simulink model "simulink_ascent_model_variable_mass_displayorganization"  (R2020a)
settings: Solver=FixedStepAuto  StartTime=0.0  StopTime=36000  FixedStep=dt  RelTol=1e-5
values from neighbouring files (symbols this model uses):
  altimeter_noise_gain = 0    [ascent_model_variable_mass.m]
  arm_tolerance = 1000    [ascent_model_variable_mass.m]
  atmo_density_noise_gain = 0    [ascent_model_variable_mass.m]
  atmo_pres_noise_gain = 0    [ascent_model_variable_mass.m]
  atmo_temp_noise_gain = 0    [ascent_model_variable_mass.m]
  burst_volume = balloon_parameters.spec.volume_burst.value    [ascent_model_variable_mass.m]
  Cd = balloon_parameters.spec.drag_coefficient    [ascent_model_variable_mass.m]
  continuous_mode = true    [ascent_model_variable_mass.m]
  delay_altitude = target_altitude    (= 24000)    [ascent_model_variable_mass.m]
  delay_time = 0    [ascent_model_variable_mass.m]
  dt = 1    [ascent_model_variable_mass.m]
  initial_altitude = 18400    [ascent_model_variable_mass.m]
  initial_velocity = 5.126    [ascent_model_variable_mass.m]
  M = molar_mass(lift_gas)    [ascent_model_variable_mass.m]    (also in molar_mass.m = 0.01604303)
  m_ballast = 0.50    (= 0.5)    [ascent_model_variable_mass.m]
  m_balloon = balloon_parameters.spec.mass.value    [ascent_model_variable_mass.m]
  m_gas_bleed = 0.50    (= 0.5)    [ascent_model_variable_mass.m]
  m_gas_reserve = 1.91    [ascent_model_variable_mass.m]
  m_payload = 2.00    (= 2)    [ascent_model_variable_mass.m]
  target_altitude = 24000    [ascent_model_variable_mass.m]
undefined symbols (not defined in the file or in its folder): m_gas
libraries: simulink x9, aerolibatmos2 x1
settings Model: Creator=Philip  LastModifiedBy=Philip
settings DataIOCC: InitialState=initial_altitude  SaveFormat=Array  SignalLogging=off  DSMLogging=off  ReturnWorkspaceOutputs=off  OutputTimes=t

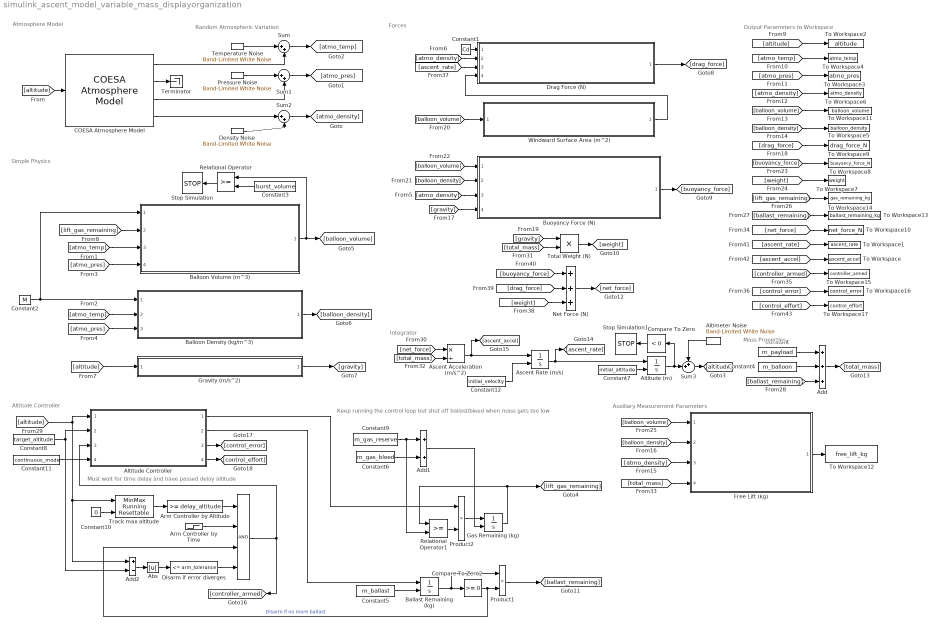
== system simulink_ascent_model_variable_mass_displayorganization ==
  note: Integrator
  note: Output Parameters to Workspace
  note: Random Atmospheric Variation
  note: Forces
  note: Simple Physics
  note: Atmosphere Model
  note: Altitude Controller
  note: Auxiliary Measurement Parameters
  note: Mass Properties
  note: Keep running the control loop but shut off ballast/bleed
      |  when mass gets too low
  note: Must wait for time delay and have passed delay altitude
  " " : Logic  Inputs=4  AllPortsSameDT=off  OutDataTypeStr=boolean
  Abs : Abs
  Add : Sum  Inputs=+++
  Add1 : Sum
  Add2 : Sum  Inputs=+-
  Altimeter Noise : simulink/Sources/Band-Limited White Noise  Cov=[altimeter_noise_gain]  Ts=dt  seed=[23341]
  Altitude (m) : Integrator  InitialConditionSource=external  InitialCondition=initial_altitude
  Altitude Controller : Subsystem  ReferencedSubsystem=altitude_control
  Arm Controller by Altitude : simulink/Logic and Bit Operations/Compare To Constant  relop=>=  const=delay_altitude  OutDataTypeStr=uint8
  Arm Controller by Time : Step  Time=delay_time  SampleTime=0
  Ascent Acceleration (m/s^2) : Product  Inputs=*/
  Ascent Rate (m/s) : Integrator  InitialConditionSource=external
  Ballast Remaining (kg) : Integrator  InitialConditionSource=external  InitialCondition=m_ballast
  Balloon Density (kg/m^3) : Subsystem  ReferencedSubsystem=rho_ideal
  Balloon Volume (m^3) : Subsystem  ReferencedSubsystem=V_ideal
  Buoyancy Force (N) : Subsystem  ReferencedSubsystem=buoyancy_force
  COESA Atmosphere Model : aerolibatmos2/COESA Atmosphere Model  units=Metric (MKS)  spec=1976 COESA-extended U.S. Standard Atmosphere  model=Profile  profile_var=High temperature  profile_percent=1%  profile_alt=5 km (16404 ft)  envelope_var=High temperature  envelope_percent=1%  action=Warning
  Compare To Zero : simulink/Logic and Bit Operations/Compare To Zero  relop=<  OutDataTypeStr=boolean
  Compare To Zero2 : simulink/Logic and Bit Operations/Compare To Zero  relop=>=  OutDataTypeStr=boolean
  Constant : Constant  Value=m_payload
  Constant1 : Constant  Value=Cd
  Constant10 : Constant  Value=0
  Constant11 : Constant  Value=continuous_mode
  Constant12 : Constant  Value=initial_velocity
  Constant2 : Constant  Value=M
  Constant3 : Constant  Value=burst_volume
  Constant4 : Constant  Value=m_balloon
  Constant5 : Constant  Value=m_ballast
  Constant6 : Constant  Value=m_gas_bleed
  Constant7 : Constant  Value=initial_altitude
  Constant8 : Constant  Value=target_altitude
  Constant9 : Constant  Value=m_gas_reserve
  Density Noise : simulink/Sources/Band-Limited White Noise  Cov=[atmo_density_noise_gain]  Ts=dt  seed=[13341]
  Disarm if error diverges : simulink/Logic and Bit Operations/Compare To Constant  relop=<=  const=arm_tolerance  OutDataTypeStr=uint8
  Drag Force (N) : Subsystem  ReferencedSubsystem=balloon_drag
  Free Lift (kg) : Subsystem  ReferencedSubsystem=free_lift
  Gas Remaining (kg) : Integrator  InitialConditionSource=external  InitialCondition=m_gas
  Gravity (m/s^2) : Subsystem  ReferencedSubsystem=gravity_simple
  Net Force (N) : Sum  Inputs=+++
  Pressure Noise : simulink/Sources/Band-Limited White Noise  Cov=[atmo_pres_noise_gain]  Ts=dt  seed=[23342]
  Product1 : Product
  Product2 : Product
  Relational Operator : RelationalOperator  OutDataTypeStr=boolean  RndMeth=Simplest
  Relational Operator1 : RelationalOperator  OutDataTypeStr=boolean  RndMeth=Simplest
  Stop Simulation : Stop
  Stop Simulation1 : Stop
  Sum : Sum  Inputs=|++
  Sum1 : Sum  Inputs=|++
  Sum2 : Sum  Inputs=|++
  Sum3 : Sum  Inputs=++|
  Temperature Noise : simulink/Sources/Band-Limited White Noise  Cov=[atmo_temp_noise_gain]  Ts=dt  seed=[23441]
  Terminator : Terminator
  To Workspace : ToWorkspace  VariableName=ascent_accel  SampleTime=-1
      settings: Save2DSignal=2-D array (concatenate along first dimension)
  To Workspace1 : ToWorkspace  VariableName=ascent_rate  SampleTime=-1
      settings: Save2DSignal=2-D array (concatenate along first dimension)
  To Workspace10 : ToWorkspace  VariableName=net_force_N  SampleTime=-1
  To Workspace11 : ToWorkspace  VariableName=balloon_volume  SampleTime=-1
  To Workspace12 : ToWorkspace  VariableName=free_lift_kg  SampleTime=-1
  To Workspace13 : ToWorkspace  VariableName=ballast_remaining_kg  SampleTime=-1
  To Workspace14 : ToWorkspace  VariableName=gas_remaining_kg  SampleTime=-1
  To Workspace15 : ToWorkspace  VariableName=controller_armed  SampleTime=-1
  To Workspace16 : ToWorkspace  VariableName=control_error  SampleTime=-1
  To Workspace17 : ToWorkspace  VariableName=control_effort  SampleTime=-1
  To Workspace2 : ToWorkspace  VariableName=altitude  SampleTime=-1
      settings: Save2DSignal=2-D array (concatenate along first dimension)
  To Workspace3 : ToWorkspace  VariableName=atmo_pres  SampleTime=-1
  To Workspace4 : ToWorkspace  VariableName=atmo_temp  SampleTime=-1
  To Workspace5 : ToWorkspace  VariableName=balloon_density  SampleTime=-1
  To Workspace6 : ToWorkspace  VariableName=atmo_density  SampleTime=-1
  To Workspace7 : ToWorkspace  VariableName=weight  SampleTime=-1
  To Workspace8 : ToWorkspace  VariableName=buoyancy_force_N  SampleTime=-1
  To Workspace9 : ToWorkspace  VariableName=drag_force_N  SampleTime=-1
  Total Weight (N) : Product
  Track max altitude : simulink/Math Operations/MinMax Running Resettable  Function=max  vinit=0.0
  Windward Surface Area (m^2) : Subsystem  ReferencedSubsystem=balloon_drag_area
  wires:
  Constant2/1 -> Balloon Density (kg/m^3)/1, Balloon Volume (m^3)/1
  COESA Atmosphere Model/3 -> Sum1/2
  Balloon Density (kg/m^3)/1 -> [balloon_density]
  Balloon Volume (m^3)/1 -> Relational Operator/1, [balloon_volume]
  Constant1/1 -> Drag Force (N)/1
  Windward Surface Area (m^2)/1 -> Drag Force (N)/4
  Relational Operator/1 -> Stop Simulation/1
  Constant3/1 -> Relational Operator/2
  Compare To Zero/1 -> Stop Simulation1/1
  Ascent Acceleration (m/s^2)/1 -> [ascent_accel], Ascent Rate (m/s)/1
  Altitude (m)/1 -> Compare To Zero/1, Sum3/2
  Buoyancy Force (N)/1 -> [buoyancy_force]
  Drag Force (N)/1 -> [drag_force]
  COESA Atmosphere Model/2 -> Terminator/1
  Gravity (m/s^2)/1 -> [gravity]
  Total Weight (N)/1 -> [weight]
  Constant/1 -> Add/1
  Ascent Rate (m/s)/1 -> Altitude (m)/1, [ascent_rate]
  Free Lift (kg)/1 -> To Workspace12/1
  Constant4/1 -> Add/2
  Constant5/1 -> Ballast Remaining (kg)/2
  Constant7/1 -> Altitude (m)/2
  Constant8/1 -> Add2/2, Altitude Controller/2
  Ballast Remaining (kg)/1 -> Product1/1, Compare To Zero2/1
  Product1/1 -> [ballast_remaining]
  Gas Remaining (kg)/1 -> Relational Operator1/1, [lift_gas_remaining]
  Altitude Controller/2 -> Ballast Remaining (kg)/1
  Arm Controller by Time/1 -> " "/2
  Arm Controller by Altitude/1 -> " "/1
  Track max altitude/1 -> Arm Controller by Altitude/1
  " "/1 -> [controller_armed], Altitude Controller/3
  Constant6/1 -> Add1/2
  Relational Operator1/1 -> Product2/2
  Constant9/1 -> Add1/1, Relational Operator1/2
  Add1/1 -> Gas Remaining (kg)/2
  Altitude Controller/1 -> Product2/1
  Product2/1 -> Gas Remaining (kg)/1
  Constant10/1 -> Track max altitude/2
  Compare To Zero2/1 -> " "/3, Product1/2  "Disarm if no more ballast"
  Sum1/1 -> [atmo_pres]
  Sum/1 -> [atmo_temp]
  Sum2/1 -> [atmo_density]
  Pressure Noise/1 -> Sum1/1
  Temperature Noise/1 -> Sum/1
  COESA Atmosphere Model/1 -> Sum/2
  COESA Atmosphere Model/4 -> Sum2/1
  Density Noise/1 -> Sum2/2
  [altitude] -> COESA Atmosphere Model/1
  [atmo_temp] -> Balloon Density (kg/m^3)/2
  [atmo_temp] -> Balloon Volume (m^3)/3
  [atmo_pres] -> Balloon Volume (m^3)/4
  [atmo_pres] -> Balloon Density (kg/m^3)/3
  [atmo_density] -> Buoyancy Force (N)/3
  [atmo_density] -> Drag Force (N)/2
  [altitude] -> Gravity (m/s^2)/1
  [lift_gas_remaining] -> Balloon Volume (m^3)/2
  [altitude] -> To Workspace2/1
  [atmo_temp] -> To Workspace4/1
  [atmo_pres] -> To Workspace3/1
  [atmo_density] -> To Workspace6/1
  [balloon_volume] -> To Workspace11/1
  [balloon_density] -> To Workspace5/1
  [atmo_density] -> Free Lift (kg)/3
  [balloon_density] -> Free Lift (kg)/2
  [gravity] -> Buoyancy Force (N)/4
  [gravity] -> Total Weight (N)/1
  [balloon_volume] -> Windward Surface Area (m^2)/1
  [balloon_density] -> Buoyancy Force (N)/2
  [balloon_volume] -> Buoyancy Force (N)/1
  [drag_force] -> To Workspace9/1
  [buoyancy_force] -> To Workspace8/1
  [weight] -> To Workspace7/1
  [balloon_volume] -> Free Lift (kg)/1
  [lift_gas_remaining] -> To Workspace14/1
  [ballast_remaining] -> To Workspace13/1
  [ballast_remaining] -> Add/3
  [altitude] -> Add2/1, Track max altitude/1, Altitude Controller/1
  Net Force (N)/1 -> [net_force]
  [net_force] -> Ascent Acceleration (m/s^2)/1
  Add/1 -> [total_mass]
  [total_mass] -> Total Weight (N)/2
  [total_mass] -> Ascent Acceleration (m/s^2)/2
  [total_mass] -> Free Lift (kg)/4
  [net_force] -> To Workspace10/1
  [ascent_rate] -> Drag Force (N)/3
  [buoyancy_force] -> Net Force (N)/1
  [drag_force] -> Net Force (N)/2
  [weight] -> Net Force (N)/3
  [ascent_rate] -> To Workspace1/1
  [ascent_accel] -> To Workspace/1
  Disarm if error diverges/1 -> " "/4
  Abs/1 -> Disarm if error diverges/1
  Add2/1 -> Abs/1
  Sum3/1 -> [altitude]
  Altimeter Noise/1 -> Sum3/1
  [controller_armed] -> To Workspace15/1
  [control_error] -> To Workspace16/1
  [control_effort] -> To Workspace17/1
  Altitude Controller/3 -> [control_error]
  Altitude Controller/4 -> [control_effort]
  Constant11/1 -> Altitude Controller/4
  Constant12/1 -> Ascent Rate (m/s)/2
